simulink model "main_simulation_without_FKw"  (R2015a)
settings: Solver=ode8  StartTime=0.0  StopTime=10  FixedStep=1e-4  RelTol=1e-3
values from neighbouring files (symbols this model uses):
  Ap = A    [main_new.m]
  At2 = Ab22-Ab21*Cb1p*Cb2    [main_new.m]
  Bp = B    [main_new.m]
  Bt2 = Bb2    [main_new.m]
  C = C(:,1:4)    [main_new.m]
  Cp = C    [main_new.m]
  Ct = M*(eye(p)-Cb1*Cb1p)*Cb2    [main_new.m]
  Gt2 = Ab21*Cb1p    [main_new.m]
  Hp = H    [main_new.m]
  Ht = M*(eye(p)-Cb1*Cb1p)    [main_new.m]
  K = Phat\Kh    [PhFunc_ga.m]    (also in main_new.m = Ph2^-1*Kh)
  L = P1^-1*Lh    [main_new.m]
  Q1 = Q(:,1:qw)    [main_new.m]
  Qbx = Q*[-Cb1p*Cb2;eye(dum6)]    [main_new.m]
  Qby = Q*[Cb1p;zeros(dum11,dum8)]    [main_new.m]
  Sai1 = Qbx*(At2-L*Ct)-A*Qbx    [main_new.m]
  Sai2 = Qbx*(Gt2+L*Ht)-A*Qby    [main_new.m]
  Sai3 = Qby    [main_new.m]
  Sai4 = Qbx*Bt2-B    [main_new.m]
  Sigma1 = Sigmaw(1:qw,:)    [main_new.m]
undefined symbols (not defined in the file or in its folder): R
libraries: simulink x3, dsparch4 x2
settings Model: Creator=p4wp4w  LastModifiedBy=p4wp4w

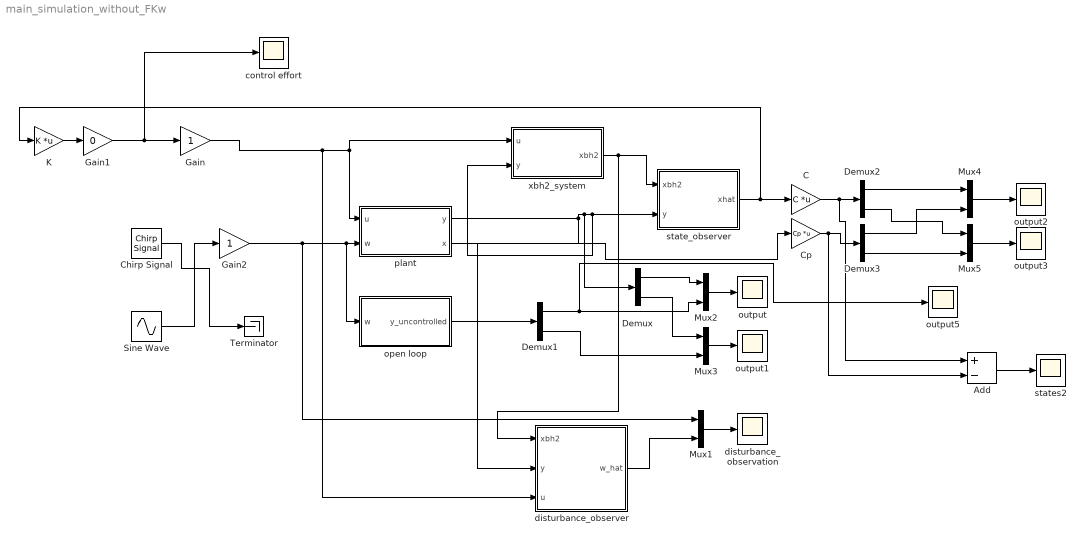
== system main_simulation_without_FKw ==
  Add : Sum  Inputs=+-
  C : Gain  Gain=C  Multiplication=Matrix(K*u)
  Chirp Signal : simulink/Sources/Chirp Signal  f1=0.1  T=10  f2=85
  Cp : Gain  Gain=Cp  Multiplication=Matrix(K*u)
  Demux{,1..3} (4 alike) : Demux  Outputs=2
  Gain : Gain
  Gain1 : Gain  Gain=0
  Gain2 : Gain
  K : Gain  Gain=K  Multiplication=Matrix(K*u)
  Mux{1..5} (5 alike) : Mux  Inputs=2
  Sine Wave : Sin  Frequency=14*2*pi  SampleTime=0
  Terminator : Terminator
  "control effort " : Scope
      settings: SaveName=ScopeData5
  disturbance_observation : Scope
      settings: SaveName=ScopeData4
  disturbance_observer : Subsystem
  open loop : Subsystem
  output{,1..3,5} (5 alike) : Scope
      output settings: YMin=-30  YMax=30
      output2 settings: YMin=-1.75  YMax=1.5  SaveName=ScopeData2
      output3 settings: SaveName=ScopeData3
      output5 settings: SaveName=ScopeData6
  plant : Subsystem
  state_observer : Subsystem
  states2 : Scope
      settings: SaveName=ScopeData7
  xbh2_system : Subsystem
  wires:
  state_observer/1(xhat) -> K/1, C/1
  plant/2(x) -> Cp/1
  xbh2_system/1(xbh2) -> disturbance_observer/1(xbh2), state_observer/1(xbh2)
  Mux1/1 -> disturbance_observation/1
  disturbance_observer/1(w_hat) -> Mux1/2
  Mux2/1 -> output/1
  Mux3/1 -> output1/1
  Demux/1 -> Mux2/1
  Demux/2 -> Mux3/1
  open loop/1(y_uncontrolled) -> Demux1/1
  Demux1/1 -> output5/1, Mux2/2
  Demux1/2 -> Mux3/2
  Gain/1 -> disturbance_observer/3(u), plant/1(u), xbh2_system/1(u)
  C/1 -> Add/1, Demux2/1
  Cp/1 -> Add/2, Demux3/1
  Demux2/1 -> Mux4/1
  Demux3/1 -> Mux4/2
  Demux2/2 -> Mux5/1
  Demux3/2 -> Mux5/2
  Mux4/1 -> output2/1
  Mux5/1 -> output3/1
  Add/1 -> states2/1
  Gain1/1 -> "control effort "/1, Gain/1
  K/1 -> Gain1/1
  plant/1(y) -> Demux/1, state_observer/2(y), xbh2_system/2(y), disturbance_observer/2(y)
  Gain2/1 -> Mux1/1, open loop/1(w), plant/2(w)
  Sine Wave/1 -> Gain2/1
  Chirp Signal/1 -> Terminator/1

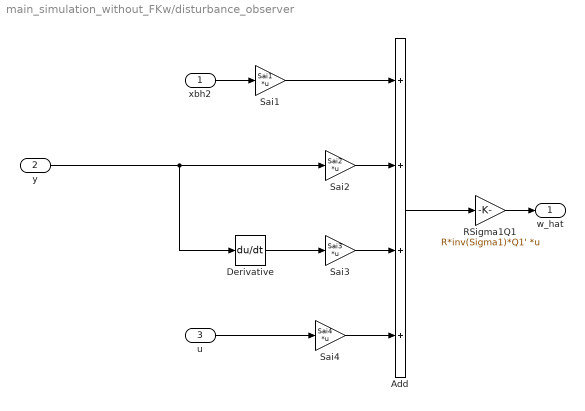
== system main_simulation_without_FKw/disturbance_observer ==
  xbh2 : Inport
  y : Inport  Port=2
  u : Inport  Port=3
  Add : Sum  Inputs=++++
  Derivative : Derivative
  RSigma1Q1 : Gain  Gain=R*inv(Sigma1)*Q1'  Multiplication=Matrix(K*u)
  Sai1 : Gain  Gain=Sai1  Multiplication=Matrix(K*u)
  Sai2 : Gain  Gain=Sai2  Multiplication=Matrix(K*u)
  Sai3 : Gain  Gain=Sai3  Multiplication=Matrix(K*u)
  Sai4 : Gain  Gain=Sai4  Multiplication=Matrix(K*u)
  w_hat : Outport
  wires:
  RSigma1Q1/1 -> w_hat/1
  Add/1 -> RSigma1Q1/1
  Sai1/1 -> Add/1
  Sai2/1 -> Add/2
  Sai3/1 -> Add/3
  Sai4/1 -> Add/4
  xbh2/1 -> Sai1/1
  y/1 -> Sai2/1, Derivative/1
  u/1 -> Sai4/1
  Derivative/1 -> Sai3/1

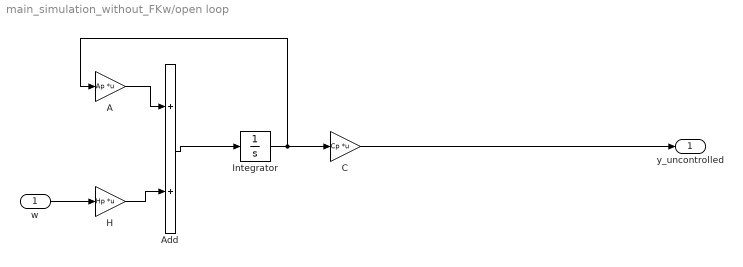
== system main_simulation_without_FKw/open loop ==
  w : Inport
  A : Gain  Gain=Ap  Multiplication=Matrix(K*u)
  Add : Sum
  C : Gain  Gain=Cp  Multiplication=Matrix(K*u)
  H : Gain  Gain=Hp  Multiplication=Matrix(K*u)
  Integrator : Integrator
  y_uncontrolled : Outport
  wires:
  C/1 -> y_uncontrolled/1
  H/1 -> Add/2
  A/1 -> Add/1
  Integrator/1 -> A/1, C/1
  Add/1 -> Integrator/1
  w/1 -> H/1

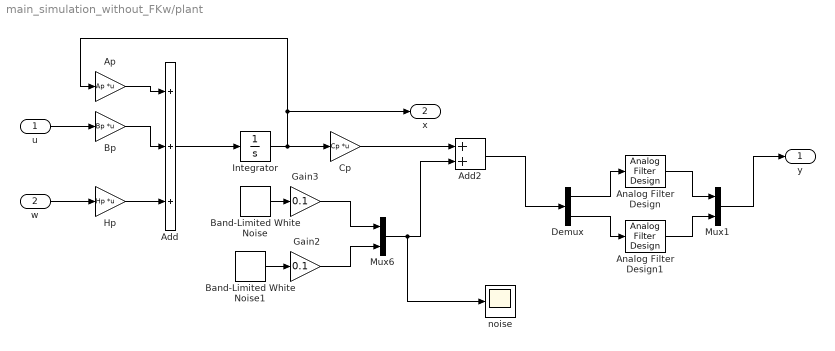
== system main_simulation_without_FKw/plant ==
  u : Inport
  w : Inport  Port=2
  Add : Sum  Inputs=+++
  Add2 : Sum
  Analog Filter Design : dsparch4/Analog Filter Design  method=Butterworth  filttype=Lowpass  N=4  Wlo=100*2*pi  Whi=80  Rp=2  Rs=40
  Analog Filter Design1 : dsparch4/Analog Filter Design  method=Butterworth  filttype=Lowpass  N=4  Wlo=100*2*pi  Whi=80  Rp=2  Rs=40
  Ap : Gain  Gain=Ap  Multiplication=Matrix(K*u)
  Band-Limited White Noise : simulink/Sources/Band-Limited White Noise  Cov=[0.000001]  Ts=1e-4  seed=[23341]
  Band-Limited White Noise1 : simulink/Sources/Band-Limited White Noise  Cov=[0.000001]  Ts=1e-4  seed=[23341]
  Bp : Gain  Gain=Bp  Multiplication=Matrix(K*u)
  Cp : Gain  Gain=Cp  Multiplication=Matrix(K*u)
  Demux : Demux  Outputs=2
  Gain2 : Gain  Gain=0.1
  Gain3 : Gain  Gain=0.1
  Hp : Gain  Gain=Hp  Multiplication=Matrix(K*u)
  Integrator : Integrator
  Mux1 : Mux  Inputs=2
  Mux6 : Mux  Inputs=2
  noise : Scope
      settings: YMin=-0.55  YMax=0.5  SaveName=ScopeData8
  y : Outport
  x : Outport  Port=2
  wires:
  w/1 -> Hp/1
  u/1 -> Bp/1
  Add/1 -> Integrator/1
  Bp/1 -> Add/2
  Integrator/1 -> Cp/1, x/1, Ap/1
  Ap/1 -> Add/1
  Hp/1 -> Add/3
  Band-Limited White Noise1/1 -> Gain2/1
  Band-Limited White Noise/1 -> Gain3/1
  Gain3/1 -> Mux6/1
  Gain2/1 -> Mux6/2
  Cp/1 -> Add2/1
  Mux6/1 -> noise/1, Add2/2
  Analog Filter Design/1 -> Mux1/1
  Analog Filter Design1/1 -> Mux1/2
  Demux/1 -> Analog Filter Design/1
  Demux/2 -> Analog Filter Design1/1
  Add2/1 -> Demux/1
  Mux1/1 -> y/1

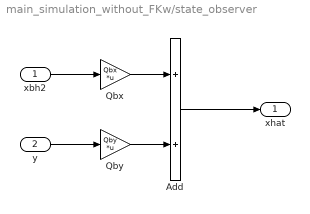
== system main_simulation_without_FKw/state_observer ==
  xbh2 : Inport
  y : Inport  Port=2
  Add : Sum
  Qbx : Gain  Gain=Qbx  Multiplication=Matrix(K*u)
  Qby : Gain  Gain=Qby  Multiplication=Matrix(K*u)
  xhat : Outport
  wires:
  Add/1 -> xhat/1
  y/1 -> Qby/1
  xbh2/1 -> Qbx/1
  Qby/1 -> Add/2
  Qbx/1 -> Add/1

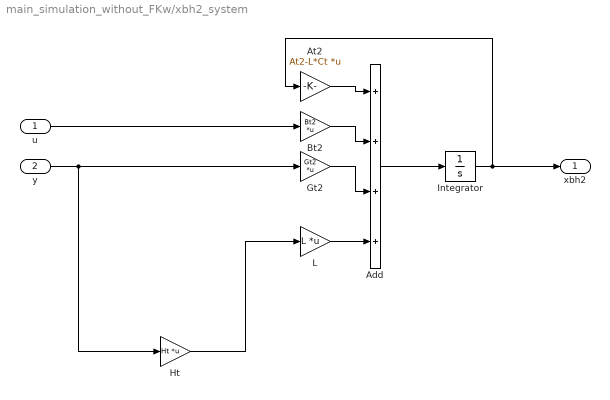
== system main_simulation_without_FKw/xbh2_system ==
  u : Inport
  y : Inport  Port=2
  Add : Sum  Inputs=++++
  At2 : Gain  Gain=At2-L*Ct  Multiplication=Matrix(K*u)
  Bt2 : Gain  Gain=Bt2  Multiplication=Matrix(K*u)
  Gt2 : Gain  Gain=Gt2  Multiplication=Matrix(K*u)
  Ht : Gain  Gain=Ht  Multiplication=Matrix(K*u)
  Integrator : Integrator
  L : Gain  Gain=L  Multiplication=Matrix(K*u)
  xbh2 : Outport
  wires:
  Gt2/1 -> Add/3
  At2/1 -> Add/1
  Integrator/1 -> xbh2/1, At2/1
  Bt2/1 -> Add/2
  Add/1 -> Integrator/1
  u/1 -> Bt2/1
  y/1 -> Ht/1, Gt2/1
  L/1 -> Add/4
  Ht/1 -> L/1
